simulink model "test1"  (R2018b)
settings: Solver=VariableStepAuto  StartTime=0.0  StopTime=10.0  RelTol=1e-3
settings Model: Creator=a4327  LastModifiedBy=a4327

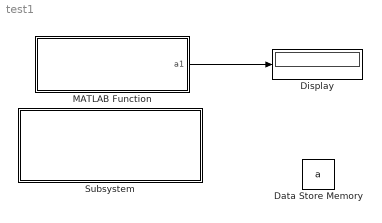
== system test1 ==
  Data Store Memory : DataStoreMemory  DataStoreName=a  ReadBeforeWriteMsg=warning  WriteAfterWriteMsg=warning  WriteAfterReadMsg=warning  ShowAdditionalParam=off  OutDataTypeStr=double
  Display : Display
  MATLAB Function : MATLAB Function  TreatAsAtomicUnit=on
  Subsystem : Subsystem
  wires:
  MATLAB Function/1(a1) -> Display/1

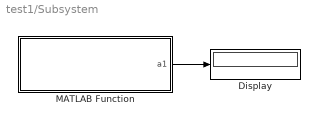
== system test1/Subsystem ==
  Display : Display
  MATLAB Function : MATLAB Function  TreatAsAtomicUnit=on
  wires:
  MATLAB Function/1(a1) -> Display/1

== matlab function test1/MATLAB Function ==
  data: a1 output; a data_store_memory
function a1=fcn
global a
a1=a;
ftest1
ftest2

== matlab function test1/Subsystem/MATLAB Function ==
  data: a1 output; a data_store_memory
function a1=fcn
global a
a1=a;
ftest1
ftest2
